simulink model "SimuPump"  (R2025a)
settings: Solver=FixedStepDiscrete  StartTime=0.0  StopTime=15  RelTol=1e-3
libraries: SignalEditorBlockLib x2
settings Model: NumberOfSteps=4  PacingRate=0.320000  Creator=moham  LastModifiedBy=moham
settings OptimizationCC: DefaultParameterBehavior=Inlined  EnhancedBackFolding=on  PassReuseOutputArgsAs=Individual arguments  ZeroExternalMemoryAtStartup=off  ZeroInternalMemoryAtStartup=off  OptimizeBlockOrder=speed  DifferentSizesBufferReuse=on  OptimizationCustomize=off  EfficientTunableParamExpr=on
settings DebuggingCC: ParameterTunabilityLossMsg=error
settings SFSimCC: MATLABDynamicMemAlloc=off
settings RTWCC: SystemTargetFile=ert.tlc  GenCodeOnly=on  TemplateMakefile=ert_default_tmf  Description=Embedded Coder
settings CodeAppCC: ForceParamTrailComments=on  IgnoreCustomStorageClasses=off  OperatorAnnotations=on  SimulinkDataObjDesc=on  SFDataObjDesc=on  InsertBlockDesc=on
settings ERTTargetCC: ExtModeTransport=0.0  ExtModeStaticAlloc=off  ExtModeMexFile=ext_comm  ExtModeIntrfLevel=Level1  ERTCustomFileTemplate=example_file_process.tlc  TargetLangStandard=C99 (ISO)  GenerateSampleERTMain=on  SupportContinuousTime=on

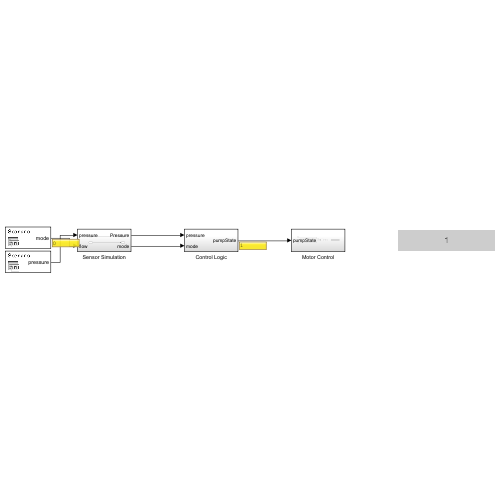
[thumbnail: Simulink's stored preview of the top-level diagram]
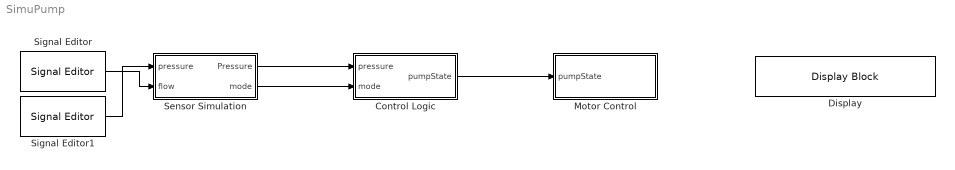
== system SimuPump ==
  Control Logic : Subsystem
  Display : DisplayBlock  LabelPosition=Hide  Transparency=1  GridColor=[0.502, 0.502, 0.502]
  Motor Control : Subsystem
  Sensor Simulation : Subsystem
  Signal Editor : SignalEditorBlockLib/Signal Editor  FileName=C:\Users\moham\SimuPumpControl\models\slprj\modeSignal.mldatx.mat  ActiveScenario=Scenario  ActiveSignal=mode  IsBus=off  OutputBusObjectStr=Bus: BusObject  SampleTime=50  ZeroCross=off  OutputAfterFinalValue=Setting to zero  Unit=inherit  PreserveSignalName=on  ApplySigPropsToAllScenarios=on  ApplySigPropsToAllSignals=off  SignalPropertySource=Dialog parameters
  Signal Editor1 : SignalEditorBlockLib/Signal Editor  FileName=C:\Users\moham\SimuPumpControl\models\slprj\pressureSignal.mldatx.mat  ActiveScenario=Scenario  ActiveSignal=pressure  IsBus=off  OutputBusObjectStr=Bus: BusObject  SampleTime=0  ZeroCross=off  OutputAfterFinalValue=Setting to zero  Unit=inherit  PreserveSignalName=on  ApplySigPropsToAllScenarios=on  ApplySigPropsToAllSignals=off  SignalPropertySource=Dialog parameters
  wires:
  Control Logic/1(pumpState) -> Motor Control/1(pumpState)
  Signal Editor1/1 -> Sensor Simulation/1(pressure)
  Signal Editor/1 -> Sensor Simulation/2(flow)
  Sensor Simulation/1(Pressure) -> Control Logic/1(pressure)
  Sensor Simulation/2(mode) -> Control Logic/2(mode)

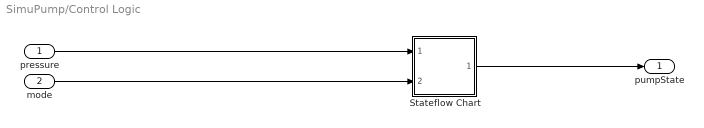
== system SimuPump/Control Logic ==
  pressure : Inport
  mode : Inport  Port=2
  " Stateflow Chart" : Stateflow chart  TreatAsAtomicUnit=on
  pumpState : Outport
  wires:
  " Stateflow Chart"/1(PumpState) -> pumpState/1
  pressure/1 -> " Stateflow Chart"/1(pressure)
  mode/1 -> " Stateflow Chart"/2(mode)

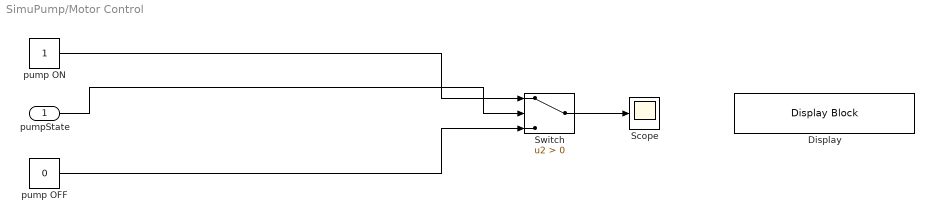
== system SimuPump/Motor Control ==
  pumpState : Inport
  Display : DisplayBlock  LabelPosition=Hide  Transparency=1  GridColor=[0.502, 0.502, 0.502]
  Scope : Scope
  Switch : Switch  Criteria=u2 > Threshold  SaturateOnIntegerOverflow=off  InputSameDT=off
  pump OFF : Constant  Value=0
  pump ON : Constant
  wires:
  pump ON/1 -> Switch/1
  pump OFF/1 -> Switch/3
  Switch/1 -> Scope/1
  pumpState/1 -> Switch/2

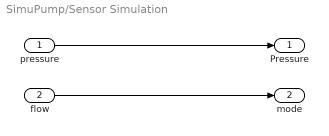
== system SimuPump/Sensor Simulation ==
  pressure : Inport
  flow : Inport  Port=2
  Pressure : Outport
  mode : Outport  Port=2
  wires:
  pressure/1 -> Pressure/1
  flow/1 -> mode/1

== stateflow chart SimuPump/Control Logic/ Stateflow Chart ==
  state Idle
    PumpState = 0;
  state Suction
    PumpState = 1;
  state Flush
    PumpState = 2;
  state Emergency
    PumpState = -1;
  (default) -> Idle
  Emergency -> Idle : [mode == 0 &&  pressure >= 0.2 || pressure <= 0.8]
  Flush -> Idle [order 3] : [mode == 0 && pressure >= 0.2 || pressure <= 0.8]
  Suction -> Idle [order 3] : [mode == 0 && pressure >= 0.2 || pressure <= 0.8]
  Idle -> Suction : [mode == 1 && pressure >= 0.2 || pressure <= 0.8]
  Flush -> Suction [order 2] : [mode == 1 && pressure >= 0.2 || pressure <= 0.8]
  Suction -> Emergency [order 2] : [pressure < 0.2 || pressure > 0.8
      | ]
  Suction -> Flush [order 1] : [mode == 2 &&  pressure >= 0.2 || pressure <= 0.8]
  Flush -> Emergency [order 1] : [pressure < 0.2 || pressure > 0.8
      | ]
  data: PumpState output double size=1; pressure input double size=1; mode input double size=1
